simulink subsystem "Battery"  (R2022a)
settings: Solver=VariableStepAuto  StartTime=0.0  StopTime=10.0  RelTol=1e-3
undefined symbols (not defined in the file or in its folder): Neg, Pos
settings Model: Creator=mateu  LastModifiedBy=mateu

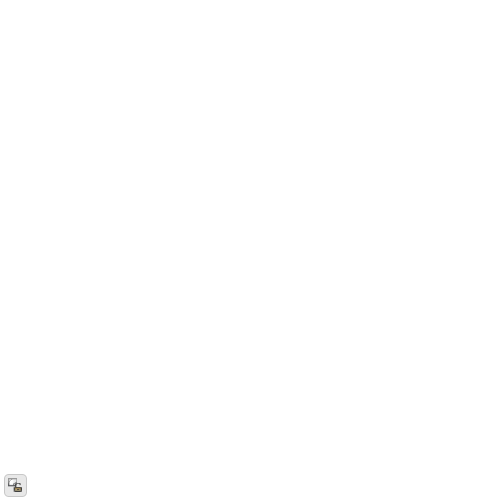
[thumbnail: Simulink's stored preview of the top-level diagram]
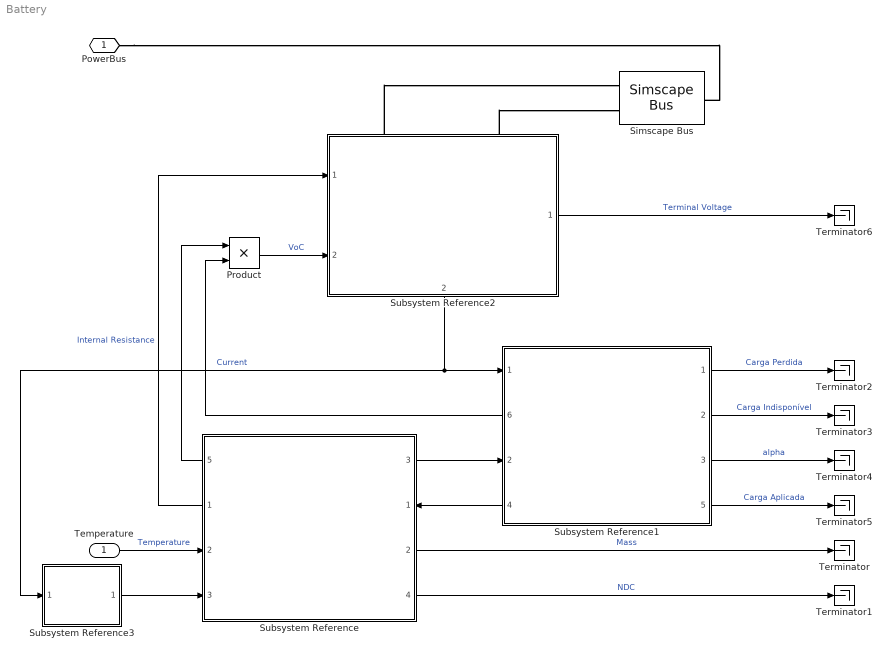
== system Battery ==
  Temperature : Inport  OutDataTypeStr=ValueType: PhysicalQuantity
  Product : Product
  Simscape Bus : SimscapeBus  HierarchyStrings=Pos;Neg  ConnectionType=Bus: DCBus
  Subsystem Reference : Subsystem  ReferencedSubsystem=Aging
      settings: PortSchema="{\"entries\":[{\"content\":{\"sides\":[{\"content\":{\"connectorIds\":[\"Out5\",\"Out1\",\"In2\",\"In3\"]},\"type\":\"ConnectorPlacement.EquallySpacedRectSide\",\"uuid\":\"07a51d5d-b148-41d7-a1ec-9d27ebf173aa\"},{\"content\":{\"connectorIds\":[\"Out3\",\"In1\",\"Out2\",\"Out4\"],\"side\":\"RIGHT\"},\"type\":\"ConnectorPlacement.EquallySpacedRectSide\",\"uuid\":\"365aca02-8db9-4b1d-92af-db486f78c2c2\"},{\"content\":{\"connectorIds\":[],\"side\":\"TOP\"},\"type\":\"ConnectorPlacement.EquallySpacedRectSide\",\"uuid\":\"da28bc68-e9ba-4965-9c22-31e867a5b626\"}]},\"type\":\"ConnectorPlacement.EquallySpacedConnector\",\"uuid\":\"4d8f8112-6e93-42b0-a312-18545d0820ca\"}],\"packageUris\":[\"http://schema.mathworks.com/mf0/Connector/R2020b\"],\"version\":\"1.0\"}"
  Subsystem Reference1 : Subsystem  ReferencedSubsystem=Diffusion
      settings: PortSchema="{\"entries\":[{\"content\":{\"sides\":[{\"content\":{\"connectorIds\":[\"In1\",\"Out6\",\"In2\",\"Out4\"]},\"type\":\"ConnectorPlacement.EquallySpacedRectSide\",\"uuid\":\"b1269a1f-65c0-4449-8281-f180240a4496\"},{\"content\":{\"connectorIds\":[\"Out1\",\"Out2\",\"Out3\",\"Out5\"],\"side\":\"RIGHT\"},\"type\":\"ConnectorPlacement.EquallySpacedRectSide\",\"uuid\":\"d4fdd221-21e4-4b96-a71e-edb41db696fb\"},{\"content\":{\"connectorIds\":[],\"side\":\"TOP\"},\"type\":\"ConnectorPlacement.EquallySpacedRectSide\",\"uuid\":\"530da0e7-f4cc-4dbe-96eb-ec2143d6abdc\"}]},\"type\":\"ConnectorPlacement.EquallySpacedConnector\",\"uuid\":\"da7f0e61-ee9a-452b-a83e-c20b4fa49ca9\"}],\"packageUris\":[\"http://schema.mathworks.com/mf0/Connector/R2020b\"],\"version\":\"1.0\"}"
  Subsystem Reference2 : Subsystem  ReferencedSubsystem=Eletrical
      settings: PortSchema="{\"entries\":[{\"content\":{\"sides\":[{\"content\":{\"connectorIds\":[\"In1\",\"In2\"]},\"type\":\"ConnectorPlacement.EquallySpacedRectSide\",\"uuid\":\"17d921fe-84ba-49b6-8165-781705691617\"},{\"content\":{\"connectorIds\":[\"Out1\"],\"side\":\"RIGHT\"},\"type\":\"ConnectorPlacement.EquallySpacedRectSide\",\"uuid\":\"2fddb0d6-aaf8-4a5b-89b9-ce64857ca82c\"},{\"content\":{\"connectorIds\":[\"LConn1\",\"LConn2\"],\"side\":\"TOP\"},\"type\":\"ConnectorPlacement.EquallySpacedRectSide\",\"uuid\":\"678dfece-e521-4f61-bcf0-145da7a3c1b5\"},{\"content\":{\"connectorIds\":[\"Out2\"],\"side\":\"BOTTOM\"},\"type\":\"ConnectorPlacement.EquallySpacedRectSide\",\"uuid\":\"098a8779-ebad-4e0b-86cc-dbdcb4374f02\"}]},\"type\":\"ConnectorPlacement.EquallySpacedConnector\",\"uuid\":\"4b2345d7-a496-4f4f-be21-c23a544cff3a\"}],\"packageUris\":[\"http://schema.mathworks.com/mf0/Connector/R2020b\"],\"version\":\"1.0\"}"
  Subsystem Reference3 : Subsystem  ReferencedSubsystem=CycleCount
  Terminator{,1..6} (7 alike) : Terminator
  PowerBus : PMIOPort  Side=Left  ConnectionType=Bus: DCBus
  wires:
  Subsystem Reference1/1 -> Terminator2/1  "Carga Perdida"
  Subsystem Reference1/3 -> Terminator4/1  "alpha"
  Subsystem Reference3/1 -> Subsystem Reference/3
  Subsystem Reference1/4 -> Subsystem Reference/1
  Subsystem Reference1/2 -> Terminator3/1  "Carga Indisponível"
  Temperature/1 -> Subsystem Reference/2  "Temperature"
  Subsystem Reference2/2 -> Subsystem Reference3/1, Subsystem Reference1/1  "Current"
  Product/1 -> Subsystem Reference2/2  "VoC"
  Subsystem Reference/4 -> Terminator1/1  "NDC"
  Subsystem Reference/2 -> Terminator/1  "Mass"
  Subsystem Reference1/5 -> Terminator5/1  "Carga Aplicada"
  Subsystem Reference1/6 -> Product/2
  Subsystem Reference/3 -> Subsystem Reference1/2
  Subsystem Reference2/1 -> Terminator6/1  "Terminal Voltage"
  Subsystem Reference/1 -> Subsystem Reference2/1  "Internal Resistance"
  Subsystem Reference/5 -> Product/1
  connections:
  PowerBus/RConn1 -- Simscape Bus/RConn1
  Subsystem Reference2/LConn1 -- Simscape Bus/LConn1
  Subsystem Reference2/LConn2 -- Simscape Bus/LConn2
